simulink model "derek_matlabModel_v3"  (R2025b)
settings: Solver=VariableStepAuto  StartTime=0.0  StopTime=5  RelTol=1e-3
values from neighbouring files (symbols this model uses):
  b = 1.53e-3    (= 0.00153)    [motorParams.m]
  J = 4.71e-4    (= 0.000471)    [motorParams.m]
  Ke = 0.257    [motorParams.m]
  Kt = Ke    (= 0.257)    [motorParams.m]
  L = Gc * P    [actualControllerProjection.m]    (also in matlabSimulations.m; motorParams.m = 0.0026; newest_matlabModel.m; open_and_closedBodePlotSims.m)
  R = 2.2    [motorParams.m]
libraries: slpidlib x1
settings Model: Creator=Derek  LastModifiedBy=Derek

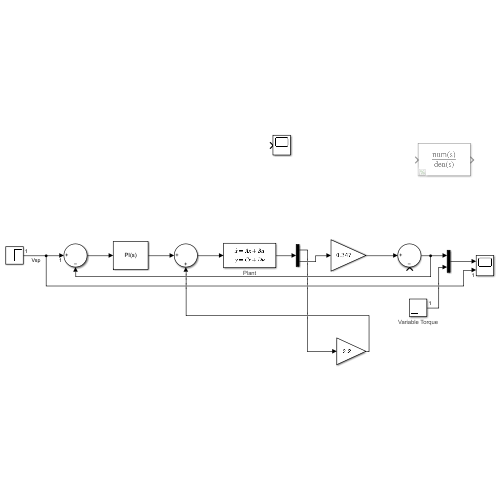
[thumbnail: Simulink's stored preview of the top-level diagram]
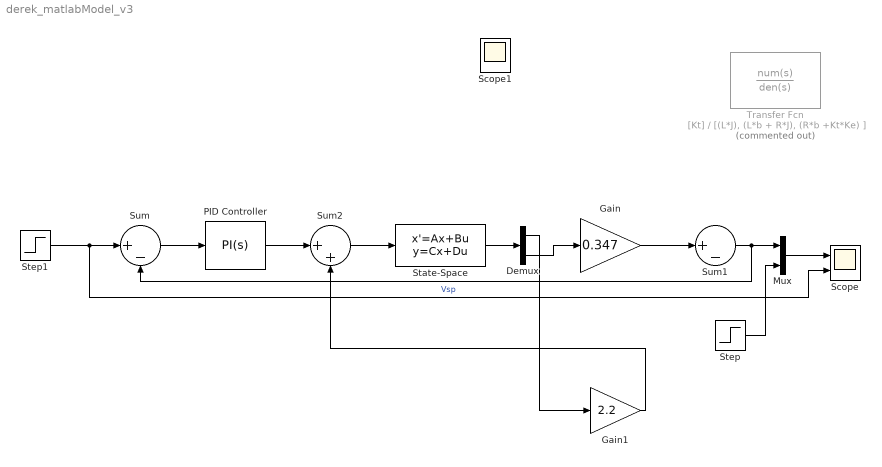
== system derek_matlabModel_v3 ==
  Demux : Demux  Outputs=2
  Gain : Gain  Gain=0.347
  Gain1 : Gain  Gain=2.2
  Mux : Mux  Inputs=2
  PID Controller : slpidlib/PID Controller  Controller=PI  Form=Parallel  TimeDomain=Continuous-time  UseExternalTs=off  SampleTime=-1  IntegratorMethod=Forward Euler  FilterMethod=Forward Euler  ControllerParametersSource=internal  P=8  I=0  UseKiTs=off  D=0  UseExternalDerivativeSource=off  N=100  UseFilter=on  TunerSelectOption=Transfer Function Based (PID Tuner App)  InitialConditionSource=internal  InitialConditionForIntegrator=0  InitialConditionForFilter=0  DifferentiatorICPrevScaledInput=0  ExternalReset=none  TrackingMode=off  Kt=1  LimitOutput=off  SatLimitsSource=internal  UpperSaturationLimit=12  LowerSaturationLimit=0  LinearizeAsGain=off  AntiWindupMode=clamping  Kb=1  LimitIntegrator=off  UpperIntegratorSaturationLimit=inf  LowerIntegratorSaturationLimit=-inf  SaturateOnIntegerOverflow=on  POutMin=[]  POutMax=[]  IOutMin=[]  IOutMax=[]  DOutMin=[]  DOutMax=[]  NOutMin=[]  NOutMax=[]  SumOutMin=[]  SumOutMax=[]  SaturationOutMin=[]  SaturationOutMax=[]  PParamMin=[]  PParamMax=[]  IParamMin=[]  IParamMax=[]  DParamMin=[]  DParamMax=[]  NParamMin=[]  NParamMax=[]  KbParamMin=[]  KbParamMax=[]  KtParamMin=[]  KtParamMax=[]  KbOutMin=[]  KbOutMax=[]  KtOutMin=[]  KtOutMax=[]  IntegratorOutMin=[]  IntegratorOutMax=[]  FilterOutMin=[]  FilterOutMax=[]  SumI1OutMin=[]  SumI1OutMax=[]  SumI2OutMin=[]  SumI2OutMax=[]  SumI3OutMin=[]  SumI3OutMax=[]  SumI4OutMin=[]  SumI4OutMax=[]  SumDOutMin=[]  SumDOutMax=[]  DifferentiatorOutMin=[]  DifferentiatorOutMax=[]  FilterDiffOutCoefMin=[]  FilterDiffOutCoefMax=[]  ReciprocalOutMin=[]  ReciprocalOutMax=[]  SumDenOutMin=[]  SumDenOutMax=[]  SumNumOutMin=[]  SumNumOutMax=[]  DivideOutMin=[]  DivideOutMax=[]  UdiffTsProdOutMin=[]  UdiffTsProdOutMax=[]  NTsProdOutMin=[]  NTsProdOutMax=[]  UintegralTsProdOutMin=[]  UintegralTsProdOutMax=[]  UngainTsProdOutMin=[]  UngainTsProdOutMax=[]  ClampingZeroOutDataTypeStr=Inherit: Inherit via back propagation  ClampingZeroOutMin=[]  ClampingZeroOutMax=[]  FilterDenConstantOutDataTypeStr=Inherit: Inherit via back propagation  FilterDenConstantOutMin=[]  FilterDenConstantOutMax=[]  PCopyOutDataTypeStr=Inherit: Inherit via back propagation  PCopyOutMin=[]  PCopyOutMax=[]  NCopyOutDataTypeStr=Inherit: Inherit via back propagation  NCopyOutMin=[]  NCopyOutMax=[]  IntegratorContinuousStateAttributes=''  IntegratorStateMustResolveToSignalObject=off  IntegratorRTWStateStorageClass=Auto  FilterContinuousStateAttributes=''  FilterStateMustResolveToSignalObject=off  FilterRTWStateStorageClass=Auto  ParallelPVariant=InternalParameters  IdealPVariant=Disabled  IVariant=InternalParameters  DVariant=Disabled  IntegratorVariant=Continuous  SatVariant=Disabled  AWVariant=Passthrough  PCopyVariant=Disabled  TRVariant=Disabled  FdbkBlocksVariant=Forward  IdealPFdbkVariant=Disabled  SatFdbkVariant=Disabled  DerivativeFilterVariant=Disabled  NVariant=Disabled  NCopyVariant=Disabled_SignalSpec  FilterICVariant=Disabled  IntegratorICVariant=InternalICs  ExternalResetVariant=Disabled  TRSumVariant=Passthrough  SumFdbkVariant=Disabled  SumVariant=Sum_PI  TsampFilterVariant=InternalTs  TsampNgainVariant=Passthrough  TsampIntegralVariant=Disabled_SignalSpec  ExternalSaturationOutDataTypeStr=Inherit: Same as second input  DerivativeSourceVariant=Disabled  PreIntVariant=InternalPreInt
  Scope : Scope  NumInputPorts=2
      settings: ActiveDisplayYMinimum=4.8116900722507934  ActiveDisplayYMaximum=6.6014564203927639
  Scope1 : Scope
      settings: ActiveDisplayYMinimum=-36.978258995223563  ActiveDisplayYMaximum=126.06336108109602
  State-Space : StateSpace  A=[-R/L -Ke/L; Kt/J -b/J]  B=[1/L 0; 0 -1/J]  C=[1 0; 0 1]  D=[0 0; 0 0]  InitialCondition=0  AllowTunableDMatrix=on
      settings: AttributesFormatString=Plant
  Step : Step  Time=0.5  SampleTime=10
      settings: AttributesFormatString=Variable Torque
  Step1 : Step  Time=2  Before=2  After=6  SampleTime=0
  Sum : Sum  Description=e = SP - PV  Inputs=|+-
  Sum1 : Sum  Description=e = SP - PV  Inputs=|+-
  Sum2 : Sum  Description=e = SP - PV  Inputs=|++
  Transfer Fcn : TransferFcn  Commented=on  Numerator=[Kt]  Denominator=[(L*J), (L*b + R*J), (R*b +Kt*Ke) ]
  wires:
  Sum/1 -> PID Controller/1
  Step1/1 -> Scope/2, Sum/1  "Vsp"
  Sum1/1 -> Sum/2, Mux/1
  Mux/1 -> Scope/1
  Step/1 -> Mux/2
  PID Controller/1 -> Sum2/1
  Gain1/1 -> Sum2/2
  Sum2/1 -> State-Space/1
  State-Space/1 -> Demux/1
  Demux/2 -> Gain/1
  Gain/1 -> Sum1/1
  Demux/1 -> Gain1/1
